simulink model "Fun"  (R2016b)
settings: Solver=FixedStepAuto  StartTime=0.0  StopTime=6  FixedStep=0.001  MaxStep=0.01  MinStep=0.01  RelTol=1e-3  EnableMultiTasking=on
libraries: aerolib6dof2 x1
settings Model: Creator=Administrator  LastModifiedBy=Administrator
settings DataIOCC: LimitDataPoints=on  SaveFormat=Array
settings OptimizationCC: LifeSpan=inf
settings DebuggingCC: UnderspecifiedInitializationDetection=Classic  MergeDetectMultiDrivingBlocksExec=none  SolverPrmCheckMsg=warning  StateNameClashWarn=warning  SFUnexpectedBacktrackingDiag=warning  SFNoUnconditionalDefaultTransitionDiag=warning  SFExecutionAtInitializationDiag=none
settings HardwareCC: ProdBitPerPointer=32  ProdBitPerSizeT=32  ProdBitPerPtrDiffT=32  ProdLargestAtomicFloat=None  ProdIntDivRoundTo=Undefined  ProdEndianess=Unspecified  ProdWordSize=32  ProdHWDeviceType=32-bit Generic
settings ModelReferenceCC: PropagateSignalLabelsOutOfModel=off
settings GRTTargetCC: TargetLangStandard=C89/C90 (ANSI)  GeneratePreprocessorConditionals=Disable all
settings ConfigComp: CovMetricSettings=dw  CovHtmlReporting=on  CovSaveCumulativeToWorkspaceVar=on  CovSaveSingleToWorkspaceVar=on  CovExternalEMLEnable=off

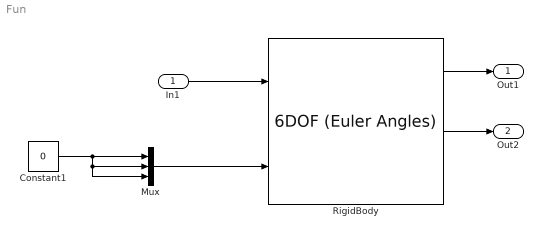
== system Fun ==
  In1 : Inport
  Constant1 : Constant  Value=0
  Mux : Mux  Inputs=3
  RigidBody : aerolib6dof2/6DOF (Euler Angles)  units=Metric (MKS)  mtype=Fixed  rep=Euler Angles  xme_0="[1  2  3]"  Vm_0=[1 2 3]  eul_0=[0 0 0]  pm_0=[ 1 1 1]  mass_0=1.0  mass_e=0.5  mass_f=2.0  inertia=eye(3)*123  inertia_e=eye(3)  inertia_f=2*eye(3)  k_quat=1.0  vre_flag=on
  Out1 : Outport
  Out2 : Outport  Port=2
  wires:
  Constant1/1 -> Mux/3, Mux/2, Mux/1
  In1/1 -> RigidBody/1
  Mux/1 -> RigidBody/2
  RigidBody/5 -> Out2/1
  RigidBody/2 -> Out1/1
